simulink model "ParallelNewSystem"  (R2017b)
settings: Solver=FixedStepDiscrete  StartTime=0.0  StopTime=17  FixedStep=0.01  RelTol=1e-3
InitFcn:
  | ra = 4;
  | jm = 0.0000218;
  | rm = 0.7/100;
  | dsm = 62.892;
  | kt = 0.138;
  | ke = kt;
  | ms = 0.93;
  | hl = 1.5 / 100;
  | Lr = 24.1 / 100;
  | Lcm = hl / 2 + Lr;
  | ml =0.182;
  | mr = 0.085;
  | rl = 20.125 / 1000;
  | Jp =1/3 * mr * Lr^2 + 1/2*ml*rl^2 + ml * Lcm ^ 2;
  | Dp = 0.007;
  | g = 9.82;
StartFcn:
  | ra = 4;
  | jm = 0.0000218;
  | rm = 0.7/100;
  | dsm = 62.892;
  | kt = 0.138;
  | ke = kt;
  | ms = 0.93;
undefined symbols (not defined in the file): PKi, PKp, setPoint, SKi, SKp
libraries: simulink x2
settings Model: Creator=labadmin  LastModifiedBy=labadmin
settings RTWCC: SystemTargetFile=sldrt.tlc  TemplateMakefile=sldrt.tmf  Description=Simulink Desktop Real-Time  RTWCompilerOptimization=on
settings CodeAppCC: MaxIdLength=95
settings SimulinkDesktopRealTimeCC: TargetPreCompLibLocation=C:\Program Files\MATLAB\R2017b\toolbox\sldrt\lib\win64

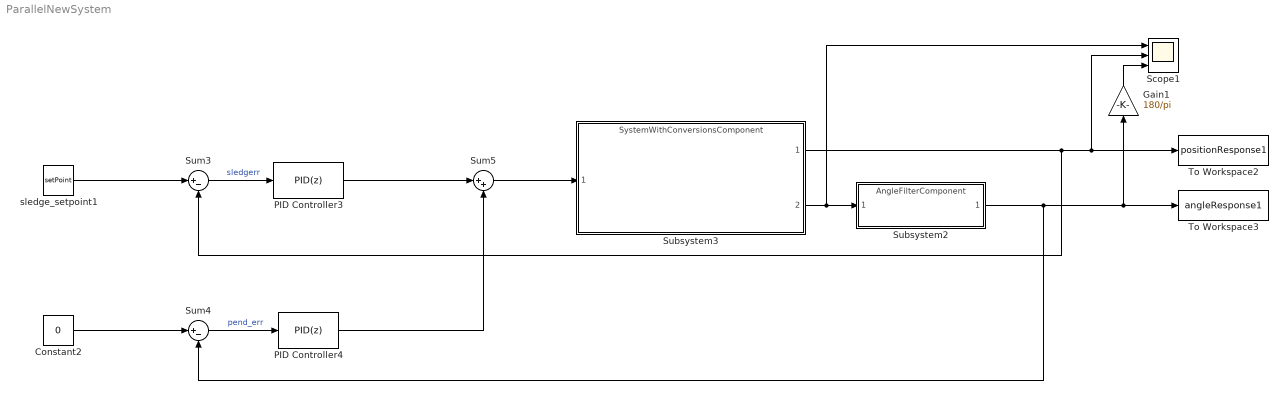
== system ParallelNewSystem ==
  Constant2 : Constant  Value=0
  Gain1 : Gain  Gain=180/pi
  PID Controller3 : simulink/Continuous/PID Controller  Controller=PID  TimeDomain=Discrete-time  SampleTime=-1  IntegratorMethod=Forward Euler  FilterMethod=Forward Euler  Form=Parallel  UseFilter=on  ControllerParametersSource=internal  P=SKp  I=SKi  D=0  N=100  InitialConditionSource=internal  InitialConditionForIntegrator=0  InitialConditionForFilter=0  ExternalReset=none  LimitOutput=off  UpperSaturationLimit=6-1.4  LowerSaturationLimit=-6+1.4  LinearizeAsGain=on  AntiWindupMode=none  Kb=1  TrackingMode=off  Kt=1  PParamMin=[]  PParamMax=[]  IParamMin=[]  IParamMax=[]  DParamMin=[]  DParamMax=[]  NParamMin=[]  NParamMax=[]  KbParamMin=[]  KbParamMax=[]  KtParamMin=[]  KtParamMax=[]  POutMin=[]  POutMax=[]  IOutMin=[]  IOutMax=[]  DOutMin=[]  DOutMax=[]  NOutMin=[]  NOutMax=[]  KbOutMin=[]  KbOutMax=[]  KtOutMin=[]  KtOutMax=[]  IntegratorOutMin=[]  IntegratorOutMax=[]  FilterOutMin=[]  FilterOutMax=[]  SumOutMin=[]  SumOutMax=[]  SumI1OutMin=[]  SumI1OutMax=[]  SumI2OutMin=[]  SumI2OutMax=[]  SumI3OutMin=[]  SumI3OutMax=[]  SumDOutMin=[]  SumDOutMax=[]  SaturationOutMin=[]  SaturationOutMax=[]  IntegratorContinuousStateAttributes=''  IntegratorStateMustResolveToSignalObject=off  IntegratorRTWStateStorageClass=Auto  FilterContinuousStateAttributes=''  FilterStateMustResolveToSignalObject=off  FilterRTWStateStorageClass=Auto  DifferentiatorICPrevScaledInput=0  DifferentiatorOutMin=[]  DifferentiatorOutMax=[]  InitialConditionSetting=State (most efficient)  FilterDiffOutCoefMin=[]  FilterDiffOutCoefMax=[]  SumDenOutMin=[]  SumDenOutMax=[]  SumNumOutMin=[]  SumNumOutMax=[]  ReciprocalOutMin=[]  ReciprocalOutMax=[]  DivideOutMin=[]  DivideOutMax=[]  TunerSelectOption=Transfer Function Based (PID Tuner App)
  PID Controller4 : simulink/Continuous/PID Controller  Controller=PID  TimeDomain=Discrete-time  SampleTime=-1  IntegratorMethod=Forward Euler  FilterMethod=Forward Euler  Form=Parallel  UseFilter=off  ControllerParametersSource=internal  P=PKp  I=PKi  D=2  N=100  InitialConditionSource=internal  InitialConditionForIntegrator=0  InitialConditionForFilter=0  ExternalReset=none  LimitOutput=off  UpperSaturationLimit=inf  LowerSaturationLimit=-inf  LinearizeAsGain=on  AntiWindupMode=none  Kb=1  TrackingMode=off  Kt=1  PParamMin=[]  PParamMax=[]  IParamMin=[]  IParamMax=[]  DParamMin=[]  DParamMax=[]  NParamMin=[]  NParamMax=[]  KbParamMin=[]  KbParamMax=[]  KtParamMin=[]  KtParamMax=[]  POutMin=[]  POutMax=[]  IOutMin=[]  IOutMax=[]  DOutMin=[]  DOutMax=[]  NOutMin=[]  NOutMax=[]  KbOutMin=[]  KbOutMax=[]  KtOutMin=[]  KtOutMax=[]  IntegratorOutMin=[]  IntegratorOutMax=[]  FilterOutMin=[]  FilterOutMax=[]  SumOutMin=[]  SumOutMax=[]  SumI1OutMin=[]  SumI1OutMax=[]  SumI2OutMin=[]  SumI2OutMax=[]  SumI3OutMin=[]  SumI3OutMax=[]  SumDOutMin=[]  SumDOutMax=[]  SaturationOutMin=[]  SaturationOutMax=[]  IntegratorContinuousStateAttributes=''  IntegratorStateMustResolveToSignalObject=off  IntegratorRTWStateStorageClass=Auto  FilterContinuousStateAttributes=''  FilterStateMustResolveToSignalObject=off  FilterRTWStateStorageClass=Auto  DifferentiatorICPrevScaledInput=0  DifferentiatorOutMin=[]  DifferentiatorOutMax=[]  InitialConditionSetting=State (most efficient)  FilterDiffOutCoefMin=[]  FilterDiffOutCoefMax=[]  SumDenOutMin=[]  SumDenOutMax=[]  SumNumOutMin=[]  SumNumOutMax=[]  ReciprocalOutMin=[]  ReciprocalOutMax=[]  DivideOutMin=[]  DivideOutMax=[]  TunerSelectOption=Transfer Function Based (PID Tuner App)
  Scope1 : Scope  NumInputPorts=3
  Subsystem2 : ModelReference  ModelNameDialog=AngleFilterComponent  SimulationMode=Normal  ModelReferenceVersion=1.19
  Subsystem3 : ModelReference  ModelNameDialog=SystemWithConversionsComponent  SimulationMode=Normal  ModelReferenceVersion=1.13
  Sum3 : Sum  Inputs=|+-
  Sum4 : Sum  Inputs=|+-
  Sum5 : Sum  Inputs=|++
  To Workspace2 : ToWorkspace  VariableName=positionResponse1  SaveFormat=Timeseries  SampleTime=-1
  To Workspace3 : ToWorkspace  VariableName=angleResponse1  SaveFormat=Timeseries  SampleTime=-1
  sledge_setpoint1 : Constant  Value=setPoint
  wires:
  Subsystem3/2 -> Scope1/1, Subsystem2/1
  Subsystem2/1 -> Sum4/2, Gain1/1, To Workspace3/1
  Constant2/1 -> Sum4/1
  PID Controller3/1 -> Sum5/1
  Sum4/1 -> PID Controller4/1  "pend_err"
  PID Controller4/1 -> Sum5/2
  Gain1/1 -> Scope1/3
  Sum3/1 -> PID Controller3/1  "sledgerr"
  Subsystem3/1 -> Scope1/2, To Workspace2/1, Sum3/2
  sledge_setpoint1/1 -> Sum3/1
  Sum5/1 -> Subsystem3/1
